simulink model "FMU_torque_vectoring6_try_antispin"  (R2023b)
settings: Solver=VariableStepAuto  StartTime=0.0  StopTime=50  RelTol=1e-3
values from neighbouring files (symbols this model uses):
  g = 9.8    [SetVehicleParameters.m]    (also in SetVehicleParameters2.m; SetVehicleParameters4.m; SetVehicleParameters5.m; SetVehicleParameters6.m)
  gearRatio = 7    [SetVehicleParameters2.m]    (also in SetVehicleParameters4.m; SetVehicleParameters5.m; SetVehicleParameters6.m)
  L = Lf + Lr    (= 3)    [SetVehicleParameters.m]    (also in SetVehicleParameters2.m = 2; SetVehicleParameters4.m = 2; SetVehicleParameters5.m = 2; SetVehicleParameters6.m = 2)
  Lr = 1.6    [SetVehicleParameters.m]    (also in SetVehicleParameters2.m = 0.5; SetVehicleParameters4.m = 0.5; SetVehicleParameters5.m = 0.5; SetVehicleParameters6.m = 0.5)
  rearTrackWidth = 1.4    [SetVehicleParameters.m]    (also in SetVehicleParameters2.m = 1; SetVehicleParameters4.m = 1; SetVehicleParameters5.m = 1; SetVehicleParameters6.m = 1)
  wheelRadiusL = 0.28    [SetVehicleParameters4.m]    (also in SetVehicleParameters5.m; SetVehicleParameters6.m)
libraries: slpidlib x3, commblkintrlv2 x1, vehdynlibviscommon x1, SignalEditorBlockLib x1, matrix_library x1
settings Model: Creator=denoc  LastModifiedBy=denoc

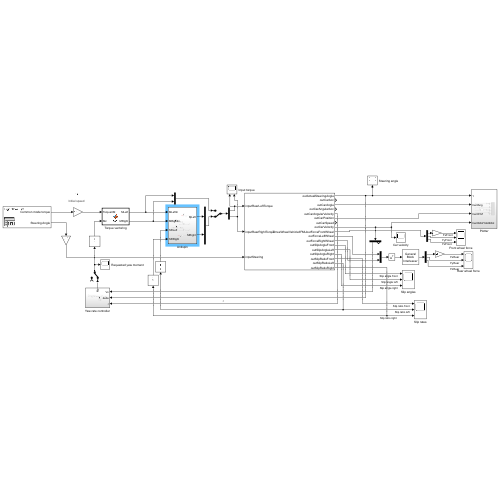
[thumbnail: Simulink's stored preview of the top-level diagram]
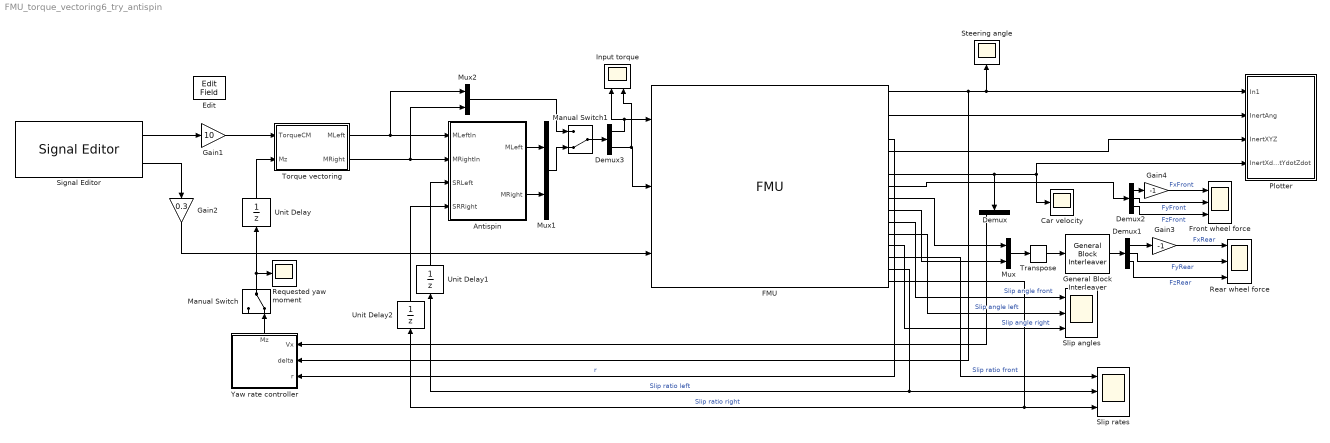
== system FMU_torque_vectoring6_try_antispin ==
  Antispin : Subsystem
  Car velocity : Scope
  Demux : Demux  Outputs=2
  Demux1 : Demux  Outputs=3
  Demux2 : Demux  Outputs=3
  Demux3 : Demux  Outputs=2
  Edit : EditField  LabelPosition=Hide  ShowInitialText=on  Alignment=Center
      settings: AttributesFormatString=Initial speed
  FMU : FMU  FMUName=ThreeWheelVehicle3FMU.fmu  FMUMode=ModelExchange  FMUInitializeEnumObject=off  FMUCachedDialogLayout="{\"Geometry\":[468,174,698,530],\"ParameterColumnsWidthConfig\":\"{\\\"columns\\\":[{\\\"name\\\":\\\"Parameter\\\",\\\"width\\\":282},{\\\"name\\\":\\\"Value\\\",\\\"width\\\":237},{\\\"name\\\":\\\"Unit\\\",\\\"width\\\":225},{\\\"name\\\":\\\"Description\\\",\\\"width\\\":293}]}\",\"InputColumnsWidthConfig\":[],\"OutputColumnsWidthConfig\":\"{\\\"columns\\\":[{\\\"name\\\":\\\"Name\\\",\\\"width\\\":287},{\\\"name\\\":\\\"Visibility\\\",\\\"width\\\":79},{\\\"name\\\":\\\"Start\\\",\\\"width\\\":137},{\\\"name\\\":\\\"Unit\\\",\\\"width\\\":134},{\\\"name\\\":\\\"Type Object\\\",\\\"width\\\":190}]}\"}"  airResistanceLongitudinal=struct('r',[0.0,1.0],'rho',1.18)  backLength=Lr  body2=struct('I',1e-08,'m',0.1)  c_rollF=rollResF  c_rollL=rollResL  c_rollR=rollResR  dragCoef=dragCoeff  front=struct('r',[0.0],'width',0.2)  front2=struct('r',[1e-10,0.0])  frontLength=Lf  frontTrail=struct('r',[0.0,-0.1])  frontWheel=struct('diameter',0.1,'r',[0.0,1.0],'v0_roll',0.1)  g=g  gearRatio=gearRatio  inertiaBody=Izz  inertiaWheelF=inertiaF  inertiaWheelL=inertiaL  inertiaWheelR=inertiaR  mass=mass  massCenterZ=h  muAF=muAF  muAL=muAL  muAR=muAR  muSF=muSF  muSL=muSL  muSR=muSR  neg=struct('k',-1.0)  neg2=struct('k',-1.0)  planarWorld=struct('constantGravity',[0.0,0.0],'defaultFrameDiameterFraction',40.0,'defaultN_to_m',1000.0,'defaultNm_to_m',1000.0,'defaultSpecularCoefficient',0.7,'defaultWidthFraction',20.0,'defaultZPosition',0.0,'gravityArrowTail',[0.0,0.0],'nominalLength',1.0)  positionPhi=struct('f_crit',50.0)  rear=struct('r',[0.0],'width',0.2)  rearLeft=struct('r',[0,0.0])  rearLeftWheel=struct('diameter',0.1,'r',[0.0,1.0],'v0_roll',0.1)  rearRight=struct('r',[0,0.0])  rearRightWheel=struct('diameter',0.1,'r',[0.0,1.0],'v0_roll',0.1)  sAdF=sAdF  sAdL=sAdL  sAdR=sAdR  sSlF=sSlF  sSlL=sSlL  sSlR=sSlR  speedStart=14  turnRadiusMAX=1000.0  vAdF=vAdF  vAdL=vAdL  vAdR=vAdR  vSlF=vSlF  vSlL=vSlL  vSlR=vSlR  vehicleFrontArea=1.5  vehicleWidth=rearTrackWidth  wheelRadiusF=wheelRadiusF  wheelRadiusL=wheelRadiusL  wheelRadiusR=wheelRadiusR  body_sphere_shapeType=sphere  body2_sphere_shapeType=sphere  front_cylinder_shapeType=cylinder  front2_cylinder_shapeType=cylinder  frontTrail_cylinder_shapeType=cylinder  frontWheel_cylinder_shapeType=cylinder  frontWheel_rim1_shapeType=cylinder  frontWheel_rim2_shapeType=cylinder  planarWorld_label1=x  planarWorld_label2=y  rear_cylinder_shapeType=cylinder  rearLeft_cylinder_shapeType=cylinder  rearLeftWheel_cylinder_shapeType=cylinder  rearLeftWheel_rim1_shapeType=cylinder  rearLeftWheel_rim2_shapeType=cylinder  rearRight_cylinder_shapeType=cylinder  rearRightWheel_cylinder_shapeType=cylinder  rearRightWheel_rim1_shapeType=cylinder  rearRightWheel_rim2_shapeType=cylinder  revolute_cylinder_shapeType=cylinder  mask(ThreeWheelVehicle3FMU [Model Exchange, v2.0]){}
      settings: MultithreadedSim=off
      mask Display:
      | disp('ThreeWheelVehicle3FMU');
      | port_label('output',1,'outActualSteeringAngle');
      | port_label('output',2,'outCarAcc');
      | port_label('output',3,'outCarAngle');
      | port_label('output',4,'outCarAngularAcc');
      | port_label('output',5,'outCarAngularVelocity');
      | port_label('output',6,'outCarPosition');
      | port_label('output',7,'outCarSpeed');
      | port_label('output',8,'outCarVelocity');
      | port_label('output',9,'outForceFrontWheel');
      | port_label('output',10,'outForceLeftWheel');
      | port_label('output',11,'outForceRightWheel');
      | port_label('output',12,'outSlipAngleFront');
      | port_label('output',13,'outSlipAngleLeft');
      | port_label('output',14,'outSlipAngleRight');
      | port_label('output',15,'outSlipRatioFront');
      | port_label('output',16,'outSlipRatioLeft');
      | port_label('output',17,'outSlipRatioRight');
      | port_label('input',1,'inputRearLeftTorque');
      | port_label('input',2,'inputRearRightTorque');
      | port_label('input',3,'inputSteering');
  Front wheel force : Scope  NumInputPorts=3
  Gain1 : Gain  Gain=10
  Gain2 : Gain  Gain=0.3
  Gain3 : Gain  Gain=-1
  Gain4 : Gain  Gain=-1
  General Block Interleaver : commblkintrlv2/General Block Interleaver  StatePerturbationForJacobian=1.0e-05  permutationVectorSource=Dialog  elements=[1;4;2;5;3;6]
  Input torque : Scope  NumInputPorts=2
  Manual Switch : ManualSwitch  CurrentSetting=0
  Manual Switch1 : ManualSwitch  CurrentSetting=0
  Mux : Mux  Inputs=2
  Mux1 : Mux  Inputs=2
  Mux2 : Mux  Inputs=2
  Plotter : Subsystem
  Rear wheel force : Scope  NumInputPorts=3
  Requested yaw moment : Scope
  Signal Editor : SignalEditorBlockLib/Signal Editor  FileName=signals.mat  ActiveScenario=RightThenLeft  ActiveSignal=Steering Angle  IsBus=off  OutputBusObjectStr=Bus: BusObject  SampleTime=0  ZeroCross=off  OutputAfterFinalValue=Holding final value  Unit=inherit  PreserveSignalName=on  ApplySigPropsToAllScenarios=on  ApplySigPropsToAllSignals=on
  Slip angles : Scope  NumInputPorts=3
  Slip rates : Scope  NumInputPorts=3
  Steering angle : Scope
  Torque vectoring : MATLAB Function  TreatAsAtomicUnit=on
  Transpose : matrix_library/Transpose
  Unit Delay : UnitDelay  SampleTime=0.001  HasFrameUpgradeWarning=on
  Unit Delay1 : UnitDelay  SampleTime=-1  HasFrameUpgradeWarning=on
  Unit Delay2 : UnitDelay  SampleTime=-1  HasFrameUpgradeWarning=on
  Yaw rate controller : Subsystem
      settings: PortSchema="{\"entries\":[{\"content\":{\"sides\":[{\"content\":{},\"type\":\"ConnectorPlacement.EquallySpacedRectSide\",\"uuid\":\"857998bb-17b2-4c26-a88e-7a272ab33241\"},{\"content\":{\"connectorIds\":[\"In1\",\"In2\",\"In3\"],\"side\":\"RIGHT\"},\"type\":\"ConnectorPlacement.EquallySpacedRectSide\",\"uuid\":\"e6bac797-4ab7-4d5a-9049-404e840be7e3\"},{\"content\":{\"connectorIds\":[\"Out1\"],\"side\":\"TOP\"},\"type\":\"ConnectorPlacement.EquallySpacedRectSide\",\"uuid\":\"452e310b-aafe-4970-ab47-27f3c9e5aadb\"}]},\"type\":\"ConnectorPlacement.EquallySpacedConnector\",\"uuid\":\"c70c4af1-0cf8-460a-ae4f-0fb1bd9e22f3\"}],\"packageUris\":[\"http://schema.mathworks.com/mf0/Connector/R2020b\"],\"version\":\"1.0\"}"
  wires:
  Signal Editor/2 -> Gain2/1
  Signal Editor/1 -> Gain1/1
  Gain2/1 -> FMU/3
  FMU/3 -> Plotter/2(InertAng)
  FMU/6 -> Plotter/3(InertXYZ)
  FMU/8 -> Car velocity/1, Plotter/4(InertXdotYdotZdot), Demux/1
  Demux/1 -> Yaw rate controller/1(Vx)
  Yaw rate controller/1(Mz) -> Manual Switch/2
  Manual Switch/1 -> Requested yaw moment/1, Unit Delay/1
  Gain1/1 -> Torque vectoring/1(TorqueCM)
  Unit Delay/1 -> Torque vectoring/2(Mz)
  FMU/5 -> Yaw rate controller/3(r)  "r"
  FMU/10 -> Mux/1
  FMU/11 -> Mux/2
  FMU/1 -> Yaw rate controller/2(delta), Steering angle/1, Plotter/1(In1)
  General Block Interleaver/1 -> Demux1/1
  Demux1/1 -> Gain3/1
  Demux1/2 -> Rear wheel force/2  "FyRear"
  Demux1/3 -> Rear wheel force/3  "FzRear"
  Mux/1 -> Transpose/1
  Transpose/1 -> General Block Interleaver/1
  Gain3/1 -> Rear wheel force/1  "FxRear"
  Demux2/1 -> Gain4/1
  Demux2/2 -> Front wheel force/2  "FyFront"
  Demux2/3 -> Front wheel force/3  "FzFront"
  FMU/9 -> Demux2/1
  Gain4/1 -> Front wheel force/1  "FxFront"
  FMU/12 -> Slip angles/1  "Slip angle front"
  FMU/13 -> Slip angles/2  "Slip angle left"
  FMU/14 -> Slip angles/3  "Slip angle right"
  FMU/15 -> Slip rates/1  "Slip ratio front"
  FMU/16 -> Unit Delay1/1, Slip rates/2  "Slip ratio left"
  FMU/17 -> Unit Delay2/1, Slip rates/3  "Slip ratio right"
  Torque vectoring/1(MLeft) -> Mux2/1, Antispin/1(MLeftIn)
  Torque vectoring/2(MRight) -> Mux2/2, Antispin/2(MRightIn)
  Unit Delay1/1 -> Antispin/3(SRLeft)
  Unit Delay2/1 -> Antispin/4(SRRight)
  Antispin/1(MLeft) -> Mux1/1
  Antispin/2(MRight) -> Mux1/2
  Mux1/1 -> Manual Switch1/2
  Manual Switch1/1 -> Demux3/1
  Demux3/1 -> Input torque/1, FMU/1
  Demux3/2 -> Input torque/2, FMU/2
  Mux2/1 -> Manual Switch1/1

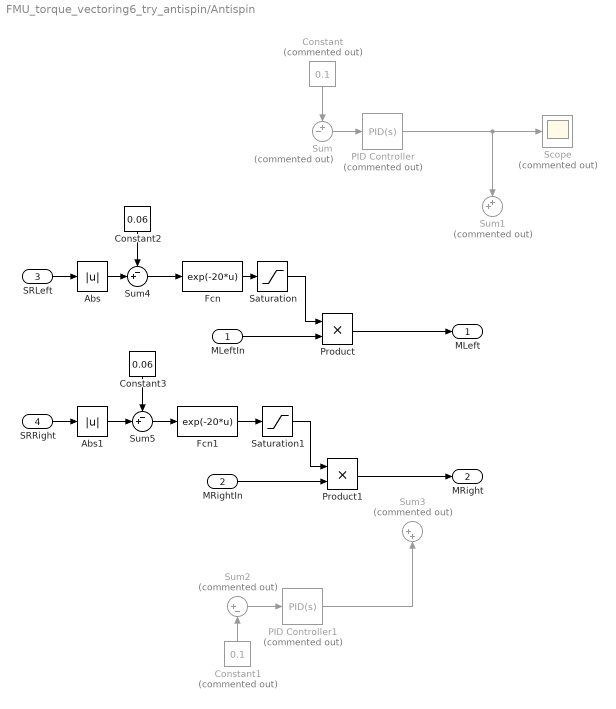
== system FMU_torque_vectoring6_try_antispin/Antispin ==
  MLeftIn : Inport
  MRightIn : Inport  Port=2
  SRLeft : Inport  Port=3
  SRRight : Inport  Port=4
  Abs : Abs  SaturateOnIntegerOverflow=off
  Abs1 : Abs  SaturateOnIntegerOverflow=off
  Constant : Constant  Commented=on  Value=0.1
  Constant1 : Constant  Commented=on  Value=0.1
  Constant2 : Constant  Value=0.06
  Constant3 : Constant  Value=0.06
  Fcn : Fcn  Expr=exp(-20*u)
  Fcn1 : Fcn  Expr=exp(-20*u)
  PID Controller : slpidlib/PID Controller  Commented=on  Controller=PID  Form=Parallel  TimeDomain=Continuous-time  UseExternalTs=off  SampleTime=-1  IntegratorMethod=Forward Euler  FilterMethod=Forward Euler  ControllerParametersSource=internal  P=0  I=5  UseKiTs=off  D=0  N=100  UseFilter=on  TunerSelectOption=Transfer Function Based (PID Tuner App)  InitialConditionSource=internal  InitialConditionForIntegrator=0  InitialConditionForFilter=0  DifferentiatorICPrevScaledInput=0  ExternalReset=none  TrackingMode=off  Kt=1  LimitOutput=on  SatLimitsSource=internal  UpperSaturationLimit=0  LowerSaturationLimit=-inf  LinearizeAsGain=on  AntiWindupMode=clamping  Kb=1  LimitIntegrator=off  UpperIntegratorSaturationLimit=inf  LowerIntegratorSaturationLimit=-inf  POutMin=[]  POutMax=[]  IOutMin=[]  IOutMax=[]  DOutMin=[]  DOutMax=[]  NOutMin=[]  NOutMax=[]  SumOutMin=[]  SumOutMax=[]  SaturationOutMin=[]  SaturationOutMax=[]  PParamMin=[]  PParamMax=[]  IParamMin=[]  IParamMax=[]  DParamMin=[]  DParamMax=[]  NParamMin=[]  NParamMax=[]  KbParamMin=[]  KbParamMax=[]  KtParamMin=[]  KtParamMax=[]  KbOutMin=[]  KbOutMax=[]  KtOutMin=[]  KtOutMax=[]  IntegratorOutMin=[]  IntegratorOutMax=[]  FilterOutMin=[]  FilterOutMax=[]  SumI1OutMin=[]  SumI1OutMax=[]  SumI2OutMin=[]  SumI2OutMax=[]  SumI3OutMin=[]  SumI3OutMax=[]  SumI4OutMin=[]  SumI4OutMax=[]  SumDOutMin=[]  SumDOutMax=[]  DifferentiatorOutMin=[]  DifferentiatorOutMax=[]  FilterDiffOutCoefMin=[]  FilterDiffOutCoefMax=[]  ReciprocalOutMin=[]  ReciprocalOutMax=[]  SumDenOutMin=[]  SumDenOutMax=[]  SumNumOutMin=[]  SumNumOutMax=[]  DivideOutMin=[]  DivideOutMax=[]  UdiffTsProdOutMin=[]  UdiffTsProdOutMax=[]  NTsProdOutMin=[]  NTsProdOutMax=[]  UintegralTsProdOutMin=[]  UintegralTsProdOutMax=[]  UngainTsProdOutMin=[]  UngainTsProdOutMax=[]  ClampingZeroOutDataTypeStr=Inherit: Inherit via back propagation  ClampingZeroOutMin=[]  ClampingZeroOutMax=[]  FilterDenConstantOutDataTypeStr=Inherit: Inherit via back propagation  FilterDenConstantOutMin=[]  FilterDenConstantOutMax=[]  PCopyOutDataTypeStr=Inherit: Inherit via back propagation  PCopyOutMin=[]  PCopyOutMax=[]  NCopyOutDataTypeStr=Inherit: Inherit via back propagation  NCopyOutMin=[]  NCopyOutMax=[]  IntegratorContinuousStateAttributes=''  IntegratorStateMustResolveToSignalObject=off  IntegratorRTWStateStorageClass=Auto  FilterContinuousStateAttributes=''  FilterStateMustResolveToSignalObject=off  FilterRTWStateStorageClass=Auto  ParallelPVariant=InternalParameters  IdealPVariant=Disabled  IVariant=InternalParameters  DVariant=InternalParameters  IntegratorVariant=Continuous  SatVariant=Enabled  AWVariant=ContClampingParallel  PCopyVariant=Disabled  TRVariant=Disabled  FdbkBlocksVariant=Forward  IdealPFdbkVariant=Disabled  SatFdbkVariant=Disabled  DerivativeFilterVariant=ContFilter  NVariant=InternalParameters  NCopyVariant=Disabled  FilterICVariant=InternalICsFilter  IntegratorICVariant=InternalICs  ExternalResetVariant=Disabled  TRSumVariant=Passthrough  SumFdbkVariant=Disabled  SumVariant=Sum_PID  TsampFilterVariant=InternalTs  TsampNgainVariant=Passthrough  TsampIntegralVariant=Disabled_SignalSpec  ExternalSaturationOutDataTypeStr=Inherit: Same as second input
  PID Controller1 : slpidlib/PID Controller  Commented=on  Controller=PID  Form=Parallel  TimeDomain=Continuous-time  UseExternalTs=off  SampleTime=-1  IntegratorMethod=Forward Euler  FilterMethod=Forward Euler  ControllerParametersSource=internal  P=0  I=5  UseKiTs=off  D=0  N=100  UseFilter=on  TunerSelectOption=Transfer Function Based (PID Tuner App)  InitialConditionSource=internal  InitialConditionForIntegrator=0  InitialConditionForFilter=0  DifferentiatorICPrevScaledInput=0  ExternalReset=none  TrackingMode=off  Kt=1  LimitOutput=on  SatLimitsSource=internal  UpperSaturationLimit=0  LowerSaturationLimit=-inf  LinearizeAsGain=on  AntiWindupMode=clamping  Kb=1  LimitIntegrator=off  UpperIntegratorSaturationLimit=inf  LowerIntegratorSaturationLimit=-inf  POutMin=[]  POutMax=[]  IOutMin=[]  IOutMax=[]  DOutMin=[]  DOutMax=[]  NOutMin=[]  NOutMax=[]  SumOutMin=[]  SumOutMax=[]  SaturationOutMin=[]  SaturationOutMax=[]  PParamMin=[]  PParamMax=[]  IParamMin=[]  IParamMax=[]  DParamMin=[]  DParamMax=[]  NParamMin=[]  NParamMax=[]  KbParamMin=[]  KbParamMax=[]  KtParamMin=[]  KtParamMax=[]  KbOutMin=[]  KbOutMax=[]  KtOutMin=[]  KtOutMax=[]  IntegratorOutMin=[]  IntegratorOutMax=[]  FilterOutMin=[]  FilterOutMax=[]  SumI1OutMin=[]  SumI1OutMax=[]  SumI2OutMin=[]  SumI2OutMax=[]  SumI3OutMin=[]  SumI3OutMax=[]  SumI4OutMin=[]  SumI4OutMax=[]  SumDOutMin=[]  SumDOutMax=[]  DifferentiatorOutMin=[]  DifferentiatorOutMax=[]  FilterDiffOutCoefMin=[]  FilterDiffOutCoefMax=[]  ReciprocalOutMin=[]  ReciprocalOutMax=[]  SumDenOutMin=[]  SumDenOutMax=[]  SumNumOutMin=[]  SumNumOutMax=[]  DivideOutMin=[]  DivideOutMax=[]  UdiffTsProdOutMin=[]  UdiffTsProdOutMax=[]  NTsProdOutMin=[]  NTsProdOutMax=[]  UintegralTsProdOutMin=[]  UintegralTsProdOutMax=[]  UngainTsProdOutMin=[]  UngainTsProdOutMax=[]  ClampingZeroOutDataTypeStr=Inherit: Inherit via back propagation  ClampingZeroOutMin=[]  ClampingZeroOutMax=[]  FilterDenConstantOutDataTypeStr=Inherit: Inherit via back propagation  FilterDenConstantOutMin=[]  FilterDenConstantOutMax=[]  PCopyOutDataTypeStr=Inherit: Inherit via back propagation  PCopyOutMin=[]  PCopyOutMax=[]  NCopyOutDataTypeStr=Inherit: Inherit via back propagation  NCopyOutMin=[]  NCopyOutMax=[]  IntegratorContinuousStateAttributes=''  IntegratorStateMustResolveToSignalObject=off  IntegratorRTWStateStorageClass=Auto  FilterContinuousStateAttributes=''  FilterStateMustResolveToSignalObject=off  FilterRTWStateStorageClass=Auto  ParallelPVariant=InternalParameters  IdealPVariant=Disabled  IVariant=InternalParameters  DVariant=InternalParameters  IntegratorVariant=Continuous  SatVariant=Enabled  AWVariant=ContClampingParallel  PCopyVariant=Disabled  TRVariant=Disabled  FdbkBlocksVariant=Forward  IdealPFdbkVariant=Disabled  SatFdbkVariant=Disabled  DerivativeFilterVariant=ContFilter  NVariant=InternalParameters  NCopyVariant=Disabled  FilterICVariant=InternalICsFilter  IntegratorICVariant=InternalICs  ExternalResetVariant=Disabled  TRSumVariant=Passthrough  SumFdbkVariant=Disabled  SumVariant=Sum_PID  TsampFilterVariant=InternalTs  TsampNgainVariant=Passthrough  TsampIntegralVariant=Disabled_SignalSpec  ExternalSaturationOutDataTypeStr=Inherit: Same as second input
  Product : Product
  Product1 : Product
  Saturation : Saturate  UpperLimit=1  LowerLimit=0
  Saturation1 : Saturate  UpperLimit=1  LowerLimit=0
  Scope : Scope  Commented=on
  Sum : Sum  Commented=on  Inputs=+-|
  Sum1 : Sum  Commented=on  Inputs=++|
  Sum2 : Sum  Commented=on  Inputs=|+-
  Sum3 : Sum  Commented=on  Inputs=|++
  Sum4 : Sum  Inputs=-+|
  Sum5 : Sum  Inputs=-+|
  MLeft : Outport
  MRight : Outport  Port=2
  wires:
  MLeftIn/1 -> Product/2
  Product/1 -> MLeft/1
  MRightIn/1 -> Product1/2
  Product1/1 -> MRight/1
  PID Controller/1 -> Sum1/1, Scope/1
  ? -> Sum/2
  Constant/1 -> Sum/1
  Sum/1 -> PID Controller/1
  Constant1/1 -> Sum2/2
  Sum2/1 -> PID Controller1/1
  PID Controller1/1 -> Sum3/2
  ? -> Sum2/1
  SRLeft/1 -> Abs/1
  Constant2/1 -> Sum4/1
  Sum4/1 -> Fcn/1
  Fcn/1 -> Saturation/1
  Saturation/1 -> Product/1
  Sum5/1 -> Fcn1/1
  SRRight/1 -> Abs1/1
  Constant3/1 -> Sum5/1
  Fcn1/1 -> Saturation1/1
  Saturation1/1 -> Product1/1
  Abs/1 -> Sum4/2
  Abs1/1 -> Sum5/2

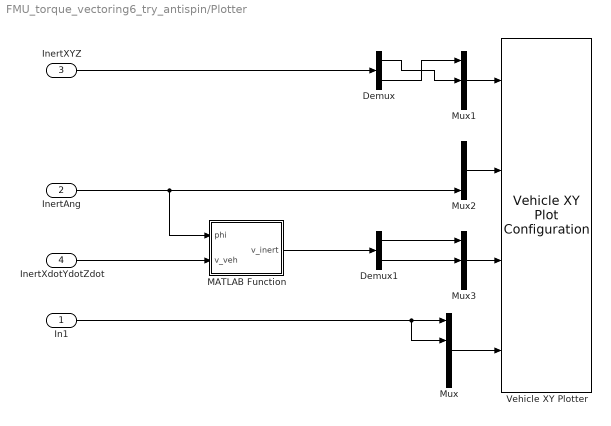
== system FMU_torque_vectoring6_try_antispin/Plotter ==
  In1 : Inport
  InertAng : Inport  Port=2
  InertXYZ : Inport  Port=3
  InertXdotYdotZdot : Inport  Port=4
  Demux : Demux  Outputs=2
  Demux1 : Demux  Outputs=2
  MATLAB Function : MATLAB Function  TreatAsAtomicUnit=on
  Mux : Mux
  Mux1 : Mux  Inputs=3
  Mux2 : Mux  Inputs=3
  Mux3 : Mux  Inputs=3
  Vehicle XY Plotter : vehdynlibviscommon/Vehicle XY Plot Configuration  extRef=off  extStats=off  extTireF=off  a=Lf  b=Lr  w=rearTrackWidth  figBorder=10  bufferSize=1024  velNorm=5  tireFNorm=1000  pltDT=.1
  wires:
  Mux/1 -> Vehicle XY Plotter/4
  Mux1/1 -> Vehicle XY Plotter/1
  Mux2/1 -> Vehicle XY Plotter/2
  InertAng/1 -> MATLAB Function/1(phi), Mux2/3
  InertXYZ/1 -> Demux/1
  Demux1/2 -> Mux3/2
  Demux1/1 -> Mux3/1
  Mux3/1 -> Vehicle XY Plotter/3
  Demux/2 -> Mux1/1
  Demux/1 -> Mux1/2
  In1/1 -> Mux/2, Mux/1
  InertXdotYdotZdot/1 -> MATLAB Function/2(v_veh)
  MATLAB Function/1(v_inert) -> Demux1/1

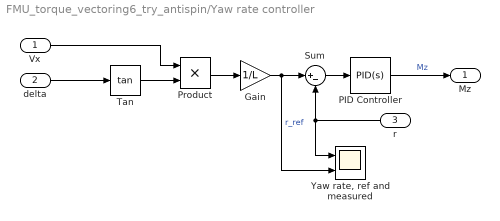
== system FMU_torque_vectoring6_try_antispin/Yaw rate controller ==
  Vx : Inport
  delta : Inport  Port=2
  r : Inport  Port=3
  Gain : Gain  Gain=1/L
  PID Controller : slpidlib/PID Controller  Controller=PID  Form=Parallel  TimeDomain=Continuous-time  UseExternalTs=off  SampleTime=-1  IntegratorMethod=Forward Euler  FilterMethod=Forward Euler  ControllerParametersSource=internal  P=700  I=180  UseKiTs=off  D=0  N=100  UseFilter=on  TunerSelectOption=Transfer Function Based (PID Tuner App)  InitialConditionSource=internal  InitialConditionForIntegrator=0  InitialConditionForFilter=0  DifferentiatorICPrevScaledInput=0  ExternalReset=none  TrackingMode=off  Kt=1  LimitOutput=off  SatLimitsSource=internal  UpperSaturationLimit=inf  LowerSaturationLimit=-inf  LinearizeAsGain=on  AntiWindupMode=none  Kb=1  LimitIntegrator=off  UpperIntegratorSaturationLimit=inf  LowerIntegratorSaturationLimit=-inf  POutMin=[]  POutMax=[]  IOutMin=[]  IOutMax=[]  DOutMin=[]  DOutMax=[]  NOutMin=[]  NOutMax=[]  SumOutMin=[]  SumOutMax=[]  SaturationOutMin=[]  SaturationOutMax=[]  PParamMin=[]  PParamMax=[]  IParamMin=[]  IParamMax=[]  DParamMin=[]  DParamMax=[]  NParamMin=[]  NParamMax=[]  KbParamMin=[]  KbParamMax=[]  KtParamMin=[]  KtParamMax=[]  KbOutMin=[]  KbOutMax=[]  KtOutMin=[]  KtOutMax=[]  IntegratorOutMin=[]  IntegratorOutMax=[]  FilterOutMin=[]  FilterOutMax=[]  SumI1OutMin=[]  SumI1OutMax=[]  SumI2OutMin=[]  SumI2OutMax=[]  SumI3OutMin=[]  SumI3OutMax=[]  SumI4OutMin=[]  SumI4OutMax=[]  SumDOutMin=[]  SumDOutMax=[]  DifferentiatorOutMin=[]  DifferentiatorOutMax=[]  FilterDiffOutCoefMin=[]  FilterDiffOutCoefMax=[]  ReciprocalOutMin=[]  ReciprocalOutMax=[]  SumDenOutMin=[]  SumDenOutMax=[]  SumNumOutMin=[]  SumNumOutMax=[]  DivideOutMin=[]  DivideOutMax=[]  UdiffTsProdOutMin=[]  UdiffTsProdOutMax=[]  NTsProdOutMin=[]  NTsProdOutMax=[]  UintegralTsProdOutMin=[]  UintegralTsProdOutMax=[]  UngainTsProdOutMin=[]  UngainTsProdOutMax=[]  ClampingZeroOutDataTypeStr=Inherit: Inherit via back propagation  ClampingZeroOutMin=[]  ClampingZeroOutMax=[]  FilterDenConstantOutDataTypeStr=Inherit: Inherit via back propagation  FilterDenConstantOutMin=[]  FilterDenConstantOutMax=[]  PCopyOutDataTypeStr=Inherit: Inherit via back propagation  PCopyOutMin=[]  PCopyOutMax=[]  NCopyOutDataTypeStr=Inherit: Inherit via back propagation  NCopyOutMin=[]  NCopyOutMax=[]  IntegratorContinuousStateAttributes=''  IntegratorStateMustResolveToSignalObject=off  IntegratorRTWStateStorageClass=Auto  FilterContinuousStateAttributes=''  FilterStateMustResolveToSignalObject=off  FilterRTWStateStorageClass=Auto  ParallelPVariant=InternalParameters  IdealPVariant=Disabled  IVariant=InternalParameters  DVariant=InternalParameters  IntegratorVariant=Continuous  SatVariant=Disabled  AWVariant=Passthrough  PCopyVariant=Disabled  TRVariant=Disabled  FdbkBlocksVariant=Forward  IdealPFdbkVariant=Disabled  SatFdbkVariant=Disabled  DerivativeFilterVariant=ContFilter  NVariant=InternalParameters  NCopyVariant=Disabled  FilterICVariant=InternalICsFilter  IntegratorICVariant=InternalICs  ExternalResetVariant=Disabled  TRSumVariant=Passthrough  SumFdbkVariant=Disabled  SumVariant=Sum_PID  TsampFilterVariant=InternalTs  TsampNgainVariant=Passthrough  TsampIntegralVariant=Disabled_SignalSpec  ExternalSaturationOutDataTypeStr=Inherit: Same as second input
  Product : Product
  Sum : Sum  Inputs=|+-
  Tan : Trigonometry  Operator=tan
  "Yaw rate, ref and measured" : Scope  NumInputPorts=2
  Mz : Outport
  wires:
  Gain/1 -> Sum/1, "Yaw rate, ref and measured"/2  "r_ref"
  PID Controller/1 -> Mz/1  "Mz"
  Sum/1 -> PID Controller/1
  r/1 -> Sum/2, "Yaw rate, ref and measured"/1
  Product/1 -> Gain/1
  Tan/1 -> Product/2
  delta/1 -> Tan/1
  Vx/1 -> Product/1

== matlab function FMU_torque_vectoring6_try_antispin/Torque vectoring ==
  data: TorqueCM input; Mz input; MLeft output; MRight output; gearRatio parameter; wheelRadiusL parameter; rearTrackWidth parameter
function [MLeft, MRight] = fcn(TorqueCM, Mz, gearRatio, wheelRadiusL, rearTrackWidth)

MDiff = wheelRadiusL * Mz / (gearRatio * rearTrackWidth);
MLeft = TorqueCM + MDiff;
MRight = TorqueCM - MDiff;

== matlab function FMU_torque_vectoring6_try_antispin/Plotter/MATLAB Function ==
  data: phi input; v_veh input; v_inert output
function v_inert  = fcn(phi, v_veh)

R = [cos(phi), -sin(phi); 
     sin(phi), cos(phi)];

v_inert = R * v_veh;
